simulink model "sim1"  (R2023a)
settings: Solver=VariableStepAuto  StartTime=0  StopTime=10  FixedStep=0.01  RelTol=1e-8
undefined symbols (not defined in the file or in its folder): a0, a1, dy0, y0
settings Model: Creator=vasil  LastModifiedBy=vasil

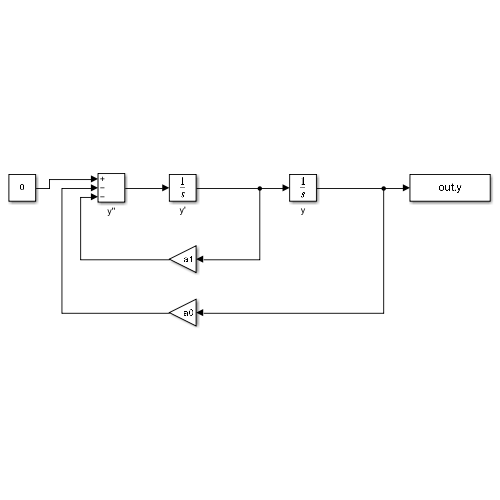
[thumbnail: Simulink's stored preview of the top-level diagram]
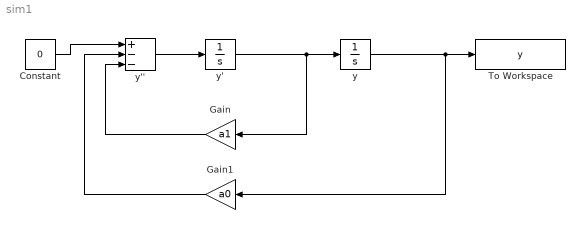
== system sim1 ==
  Constant : Constant  Value=0
  Gain : Gain  Gain=a1
  Gain1 : Gain  Gain=a0
  To Workspace : ToWorkspace  VariableName=y  SaveFormat=Timeseries  SampleTime=-1
  y : Integrator  InitialCondition=y0
  y' : Integrator  InitialCondition=dy0
  y'' : Sum  Inputs=+--
  wires:
  y/1 -> Gain1/1, To Workspace/1
  y''/1 -> y'/1
  Gain1/1 -> y''/2
  y'/1 -> Gain/1, y/1
  Constant/1 -> y''/1
  Gain/1 -> y''/3
